simulink model "ModelRobot_NEW"  (R2020a)
settings: Solver=FixedStepDiscrete  StartTime=0.0  StopTime=30  FixedStep=0.005  RelTol=1e-3
InitFcn:
  | addpath(genpath('D:\STUDY\LVTHS_NEW\mobile-robotics-simulation-toolbox-master'))
undefined symbols (not defined in the file or in its folder): sigbuilder_block
libraries: simulink x4, mcbhostblockslib x3, mobileRoboticsLib x1
settings Model: Creator=dangh  LastModifiedBy=dangh
settings DataIOCC: ReturnWorkspaceOutputsName=out1

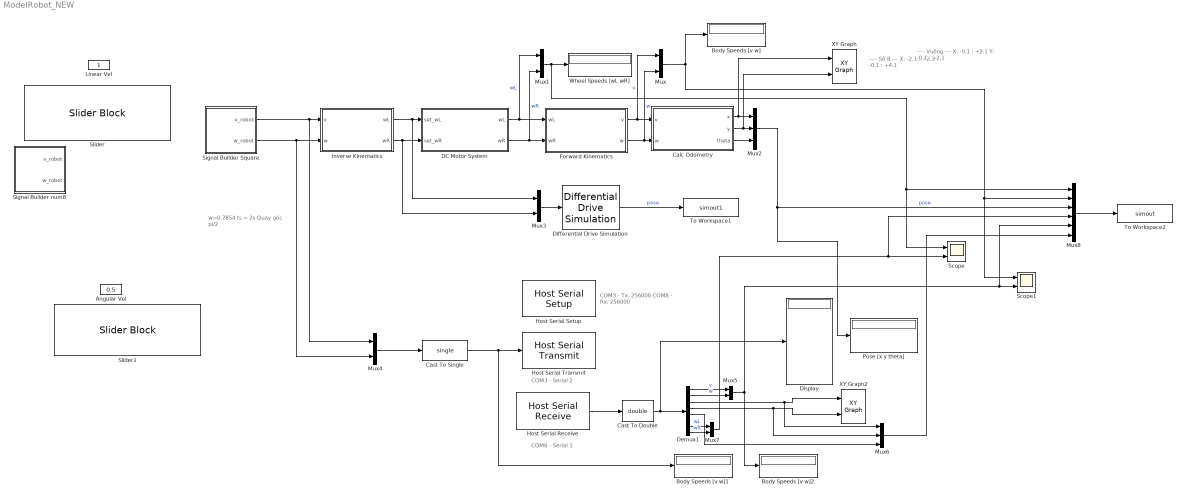
== system ModelRobot_NEW ==
  note: COM3 - Serial 2
  note: COM8 - Serial 1
  note: COM3 - Tx: 256000
      | COM8 - Rx: 256000
  note: ---- Số 8 ---
      | X: -2.1 : +2.1
      | Y: -0.1 : +4.1
  note: w=0.7854
      | ts = 2s
      | Quay góc pi/2
  note: ---- Vuông ---
      | X: -0.1 : +2.1
      | Y: -0.1 : +2.1
  Angular Vel : Constant  Value=0.5
  Body Speeds [v w] : Display
  Body Speeds [v w]1 : Display
  Body Speeds [v w]2 : Display
  Calc Odometry : MATLAB Function  TreatAsAtomicUnit=on
  Cast To Double : DataTypeConversion  OutDataTypeStr=double
  Cast To Single : DataTypeConversion  OutDataTypeStr=single
  DC Motor System : Subsystem
  Demux1 : Demux  Outputs=8
  Differential Drive Simulation : mobileRoboticsLib/Kinematic Models/Differential Drive/Differential Drive Simulation  wheelRadius=0.0625  wheelBase=0.37  initX=0  initY=0  initAngle=0  Ts=0.005
      settings: SourceProductName=Mobile Robotics Simulation Library
  Display : Display
  Forward Kinematics : MATLAB Function  TreatAsAtomicUnit=on
  Host Serial Receive : mcbhostblockslib/Host Serial Receive  serialCon=Serial 1  dataHead='S'  dataTail=0x0d  dataType=single  dataDim=8  initValue=0  errOption=Output the last received value  errValue=0  sampleTime=-1  outputStatus=off  blockingMode=off
      settings: SourceProductBaseCode=MT
  Host Serial Setup : mcbhostblockslib/Host Serial Setup  Priority=-99  comPortSer1='COM8'  baudRateA=256000  charLenA=8  stopBitA=1  parityA=none  timeoutA=1.0  ByteOrderA=LittleEndian  comPortSer2='COM3'  baudRateB=256000  charLenB=8  stopBitB=1  parityB=none  timeoutB=1.0  ByteOrderB=LittleEndian  comPortSer3='Please_select_a_port'  baudRateC=115200  charLenC=8  stopBitC=1  parityC=none  timeoutC=1.0  ByteOrderC=LittleEndian  comPortSer4='Please_select_a_port'  baudRateD=115200  charLenD=8  stopBitD=1  parityD=none  timeoutD=1.0  ByteOrderD=LittleEndian
      settings: SourceProductBaseCode=MT
  Host Serial Transmit : mcbhostblockslib/Host Serial Transmit  serialCon=Serial 2  header='S'  tail=0x0D  enableBlockingMode=off
      settings: SourceProductBaseCode=MT
  Inverse Kinematics : MATLAB Function  TreatAsAtomicUnit=on
  Linear Vel : Constant
  Mux{,1,3..5,7} (6 alike) : Mux  Inputs=2
  Mux2 : Mux  Inputs=3
  Mux6 : Mux  Inputs=3
  Mux8 : Mux  Inputs=6
  Pose [x y theta] : Display
  Scope : Scope  NumInputPorts=2
  Scope1 : Scope  NumInputPorts=2
  Signal Builder Square : Subsystem  Tag=STV Subsys  LoadFcn=sigbuilder_block('load');  StartFcn=sigbuilder_block('start');  StopFcn=sigbuilder_block('stop');  ClipboardFcn=sigbuilder_block('clipboard');  mask(Sigbuilder block){tuvar=[0:10]}
      mask help: Simulink:masks:SigbuilderBlock_MD
      mask init:
      | if ~strcmp(get_param(bdroot(gcbh),'SimulationStatus'),'stopped') tuvar = sigbuilder_block('maskInit'); end
      settings: CopyFcn=sigbuilder_block('copy');  DeleteFcn=sigbuilder_block('delete');  ModelCloseFcn=sigbuilder_block('modelClose');  PreSaveFcn=sigbuilder_block('preSave');  PauseFcn=sigbuilder_block('pause');  ContinueFcn=sigbuilder_block('continue');  NameChangeFcn=sigbuilder_block('namechange');  OpenFcn=sigbuilder_block('open',[128.25 211.5 550.5 399.75 ]);  CloseFcn=sigbuilder_block('close');
      mask Display: plot(0, 0, 100, 100,[2, 2, 32, 32, 2], [68, 8, 8, 68, 68],[32, 2], [38, 38], [32, 19, 2],[53, 60, 44], [32, 17, 17, 2],[16, 16, 31, 31]);txt = getActiveGroup(gcbh);text(2, 100, txt,'verticalAlignment', 'top');
  Signal Builder num8 : Subsystem  Tag=STV Subsys  LoadFcn=sigbuilder_block('load');  StartFcn=sigbuilder_block('start');  StopFcn=sigbuilder_block('stop');  ClipboardFcn=sigbuilder_block('clipboard');  mask(Sigbuilder block){tuvar=[0:10]}
      mask help: Simulink:masks:SigbuilderBlock_MD
      mask init:
      | if ~strcmp(get_param(bdroot(gcbh),'SimulationStatus'),'stopped') tuvar = sigbuilder_block('maskInit'); end
      settings: CopyFcn=sigbuilder_block('copy');  DeleteFcn=sigbuilder_block('delete');  ModelCloseFcn=sigbuilder_block('modelClose');  PreSaveFcn=sigbuilder_block('preSave');  PauseFcn=sigbuilder_block('pause');  ContinueFcn=sigbuilder_block('continue');  NameChangeFcn=sigbuilder_block('namechange');  OpenFcn=sigbuilder_block('open',[204 220.5 771.75 398.25 ]);  CloseFcn=sigbuilder_block('close');
      mask Display: plot(0, 0, 100, 100,[2, 2, 32, 32, 2], [68, 8, 8, 68, 68],[32, 2], [38, 38], [32, 19, 2],[53, 60, 44], [32, 17, 17, 2],[16, 16, 31, 31]);txt = getActiveGroup(gcbh);text(2, 100, txt,'verticalAlignment', 'top');
  Slider : SliderBlock  ScaleMin=-1  ScaleMax=1  TickInterval=0.25
  Slider1 : SliderBlock  ScaleMin=-1.5  ScaleMax=1.5
  To Workspace1 : ToWorkspace  VariableName=simout1  SaveFormat=Timeseries  SampleTime=-1
  To Workspace2 : ToWorkspace  VariableName=simout  SaveFormat=Timeseries  SampleTime=-1
  Wheel Speeds [wL wR] : Display
  XY Graph : simulink/Sinks/XY Graph  xmin=-2.1  xmax=2.1  ymin=-0.1  ymax=4.1  st=-1
  XY Graph2 : simulink/Sinks/XY Graph  xmin=-1  xmax=3  ymin=-2  ymax=2.5  st=-1
  wires:
  Differential Drive Simulation/1 -> To Workspace1/1  "pose"
  Inverse Kinematics/1(wL) -> DC Motor System/1(set_wL), Mux3/1
  Inverse Kinematics/2(wR) -> DC Motor System/2(set_wR), Mux3/2
  Mux/1 -> Scope1/1, Mux8/2, Body Speeds [v w]/1
  Mux1/1 -> Scope/1, Mux8/1, Wheel Speeds [wL wR]/1
  Mux3/1 -> Differential Drive Simulation/1
  DC Motor System/1(wL) -> Mux1/1, Forward Kinematics/1(wL)  "wL"
  DC Motor System/2(wR) -> Mux1/2, Forward Kinematics/2(wR)  "wR"
  Forward Kinematics/2(w) -> Mux/2, Calc Odometry/2(w)  "w"
  Forward Kinematics/1(v) -> Mux/1, Calc Odometry/1(v)  "v"
  Calc Odometry/3(theta) -> Mux2/3
  Calc Odometry/2(y) -> XY Graph/2, Mux2/2
  Calc Odometry/1(x) -> XY Graph/1, Mux2/1
  Mux2/1 -> Mux8/3, Pose [x y theta]/1  "pose"
  Mux4/1 -> Cast To Single/1
  Cast To Single/1 -> Body Speeds [v w]1/1, Host Serial Transmit/1
  Demux1/2 -> Mux5/2  "w"
  Demux1/1 -> Mux5/1  "v"
  Mux5/1 -> Mux8/5, Scope1/2, Body Speeds [v w]2/1
  Demux1/3 -> Mux6/1, XY Graph2/1
  Demux1/4 -> Mux6/2, XY Graph2/2
  Demux1/5 -> Mux6/3
  Mux6/1 -> Mux8/6
  Mux7/1 -> Mux8/4, Scope/2
  Cast To Double/1 -> Display/1, Demux1/1
  Mux8/1 -> To Workspace2/1
  Host Serial Receive/1 -> Cast To Double/1
  Signal Builder Square/2(w_robot) -> Mux4/2, Inverse Kinematics/2(w)
  Signal Builder Square/1(v_robot) -> Mux4/1, Inverse Kinematics/1(v)
  Demux1/7 -> Mux7/1  "wL"
  Demux1/8 -> Mux7/2  "wR"

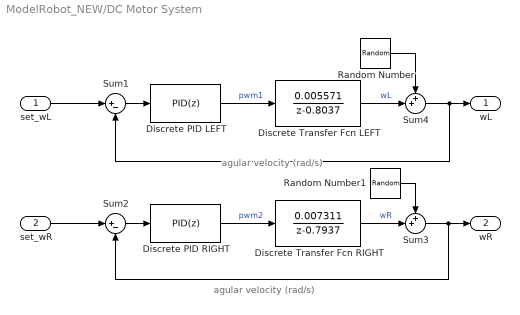
== system ModelRobot_NEW/DC Motor System ==
  note: agular velocity (rad/s)
  note: agular velocity (rad/s)
  set_wL : Inport
  set_wR : Inport  Port=2
  Discrete Transfer Fcn LEFT : DiscreteTransferFcn  Numerator=0.005571  Denominator=[1 -0.8037]
  Discrete Transfer Fcn RIGHT : DiscreteTransferFcn  Numerator=[0.007311]  Denominator=[1 -0.7937]
  Discrete PID LEFT : simulink/Continuous/PID Controller  Controller=PID  Form=Parallel  TimeDomain=Discrete-time  UseExternalTs=off  SampleTime=0.005  IntegratorMethod=Trapezoidal  FilterMethod=Forward Euler  ControllerParametersSource=internal  P=4.48920648489184  I=176.768621079225  D=0.0343896212668413  UseFilter=off  N=100  TunerSelectOption=Transfer Function Based (PID Tuner App)  InitialConditionSource=internal  InitialConditionForIntegrator=0  InitialConditionForFilter=0  DifferentiatorICPrevScaledInput=0  ExternalReset=none  TrackingMode=off  Kt=1  LimitOutput=on  UpperSaturationLimit=999  LowerSaturationLimit=-999  LinearizeAsGain=off  AntiWindupMode=none  Kb=1  POutMin=[]  POutMax=[]  IOutMin=[]  IOutMax=[]  DOutMin=[]  DOutMax=[]  NOutMin=[]  NOutMax=[]  SumOutMin=[]  SumOutMax=[]  SaturationOutMin=[]  SaturationOutMax=[]  PParamMin=[]  PParamMax=[]  IParamMin=[]  IParamMax=[]  DParamMin=[]  DParamMax=[]  NParamMin=[]  NParamMax=[]  KbParamMin=[]  KbParamMax=[]  KtParamMin=[]  KtParamMax=[]  KbOutMin=[]  KbOutMax=[]  KtOutMin=[]  KtOutMax=[]  IntegratorOutMin=[]  IntegratorOutMax=[]  FilterOutMin=[]  FilterOutMax=[]  SumI1OutMin=[]  SumI1OutMax=[]  SumI2OutMin=[]  SumI2OutMax=[]  SumI3OutMin=[]  SumI3OutMax=[]  SumI4OutMin=[]  SumI4OutMax=[]  SumDOutMin=[]  SumDOutMax=[]  DifferentiatorOutMin=[]  DifferentiatorOutMax=[]  FilterDiffOutCoefMin=[]  FilterDiffOutCoefMax=[]  ReciprocalOutMin=[]  ReciprocalOutMax=[]  SumDenOutMin=[]  SumDenOutMax=[]  SumNumOutMin=[]  SumNumOutMax=[]  DivideOutMin=[]  DivideOutMax=[]  UdiffTsProdOutMin=[]  UdiffTsProdOutMax=[]  NTsProdOutMin=[]  NTsProdOutMax=[]  UintegralTsProdOutMin=[]  UintegralTsProdOutMax=[]  UngainTsProdOutMin=[]  UngainTsProdOutMax=[]  IntegratorContinuousStateAttributes=''  IntegratorStateMustResolveToSignalObject=off  IntegratorRTWStateStorageClass=Auto  FilterContinuousStateAttributes=''  FilterStateMustResolveToSignalObject=off  FilterRTWStateStorageClass=Auto  ParallelPVariant=InternalParameters  IdealPVariant=Disabled  IVariant=InternalParameters  DVariant=InternalParameters  IntegratorVariant=Discrete  SatVariant=Enabled  AWVariant=Passthrough  PCopyVariant=Disabled  TRVariant=Disabled  FdbkBlocksVariant=Forward  IdealPFdbkVariant=Disabled  SatFdbkVariant=Disabled  DerivativeFilterVariant=Differentiator  NVariant=Passthrough  NCopyVariant=Disabled_SignalSpec  FilterICVariant=InternalICsDifferentiator  IntegratorICVariant=InternalICs  ExternalResetVariant=Disabled  TRSumVariant=Passthrough  SumFdbkVariant=Disabled  SumVariant=Sum_PID  TsampFilterVariant=InternalTs  TsampNgainVariant=Passthrough  TsampIntegralVariant=Passthrough
  Discrete PID RIGHT : simulink/Continuous/PID Controller  Controller=PID  Form=Parallel  TimeDomain=Discrete-time  UseExternalTs=off  SampleTime=0.005  IntegratorMethod=Trapezoidal  FilterMethod=Forward Euler  ControllerParametersSource=internal  P=3.42072165271296  I=141.511593847985  D=0.0251690597812978  UseFilter=off  N=100  TunerSelectOption=Transfer Function Based (PID Tuner App)  InitialConditionSource=internal  InitialConditionForIntegrator=0  InitialConditionForFilter=0  DifferentiatorICPrevScaledInput=0  ExternalReset=none  TrackingMode=off  Kt=1  LimitOutput=on  UpperSaturationLimit=999  LowerSaturationLimit=-999  LinearizeAsGain=off  AntiWindupMode=none  Kb=1  POutMin=[]  POutMax=[]  IOutMin=[]  IOutMax=[]  DOutMin=[]  DOutMax=[]  NOutMin=[]  NOutMax=[]  SumOutMin=[]  SumOutMax=[]  SaturationOutMin=[]  SaturationOutMax=[]  PParamMin=[]  PParamMax=[]  IParamMin=[]  IParamMax=[]  DParamMin=[]  DParamMax=[]  NParamMin=[]  NParamMax=[]  KbParamMin=[]  KbParamMax=[]  KtParamMin=[]  KtParamMax=[]  KbOutMin=[]  KbOutMax=[]  KtOutMin=[]  KtOutMax=[]  IntegratorOutMin=[]  IntegratorOutMax=[]  FilterOutMin=[]  FilterOutMax=[]  SumI1OutMin=[]  SumI1OutMax=[]  SumI2OutMin=[]  SumI2OutMax=[]  SumI3OutMin=[]  SumI3OutMax=[]  SumI4OutMin=[]  SumI4OutMax=[]  SumDOutMin=[]  SumDOutMax=[]  DifferentiatorOutMin=[]  DifferentiatorOutMax=[]  FilterDiffOutCoefMin=[]  FilterDiffOutCoefMax=[]  ReciprocalOutMin=[]  ReciprocalOutMax=[]  SumDenOutMin=[]  SumDenOutMax=[]  SumNumOutMin=[]  SumNumOutMax=[]  DivideOutMin=[]  DivideOutMax=[]  UdiffTsProdOutMin=[]  UdiffTsProdOutMax=[]  NTsProdOutMin=[]  NTsProdOutMax=[]  UintegralTsProdOutMin=[]  UintegralTsProdOutMax=[]  UngainTsProdOutMin=[]  UngainTsProdOutMax=[]  IntegratorContinuousStateAttributes=''  IntegratorStateMustResolveToSignalObject=off  IntegratorRTWStateStorageClass=Auto  FilterContinuousStateAttributes=''  FilterStateMustResolveToSignalObject=off  FilterRTWStateStorageClass=Auto  ParallelPVariant=InternalParameters  IdealPVariant=Disabled  IVariant=InternalParameters  DVariant=InternalParameters  IntegratorVariant=Discrete  SatVariant=Enabled  AWVariant=Passthrough  PCopyVariant=Disabled  TRVariant=Disabled  FdbkBlocksVariant=Forward  IdealPFdbkVariant=Disabled  SatFdbkVariant=Disabled  DerivativeFilterVariant=Differentiator  NVariant=Passthrough  NCopyVariant=Disabled_SignalSpec  FilterICVariant=InternalICsDifferentiator  IntegratorICVariant=InternalICs  ExternalResetVariant=Disabled  TRSumVariant=Passthrough  SumFdbkVariant=Disabled  SumVariant=Sum_PID  TsampFilterVariant=InternalTs  TsampNgainVariant=Passthrough  TsampIntegralVariant=Passthrough
  Random Number : RandomNumber  Variance=0.020583  SampleTime=0.005
  Random Number1 : RandomNumber  Variance=0.0847669  SampleTime=0.005
  Sum1 : Sum  Inputs=|+-
  Sum2 : Sum  Inputs=|+-
  Sum3 : Sum  Inputs=++|
  Sum4 : Sum  Inputs=++|
  wL : Outport
  wR : Outport  Port=2
  wires:
  Sum2/1 -> Discrete PID RIGHT/1
  Discrete PID RIGHT/1 -> Discrete Transfer Fcn RIGHT/1  "pwm2"
  set_wL/1 -> Sum1/1
  Discrete Transfer Fcn LEFT/1 -> Sum4/2  "wL"
  Sum1/1 -> Discrete PID LEFT/1
  Discrete Transfer Fcn RIGHT/1 -> Sum3/2  "wR"
  Discrete PID LEFT/1 -> Discrete Transfer Fcn LEFT/1  "pwm1"
  set_wR/1 -> Sum2/1
  Sum4/1 -> wL/1, Sum1/2
  Random Number/1 -> Sum4/1
  Random Number1/1 -> Sum3/1
  Sum3/1 -> Sum2/2, wR/1

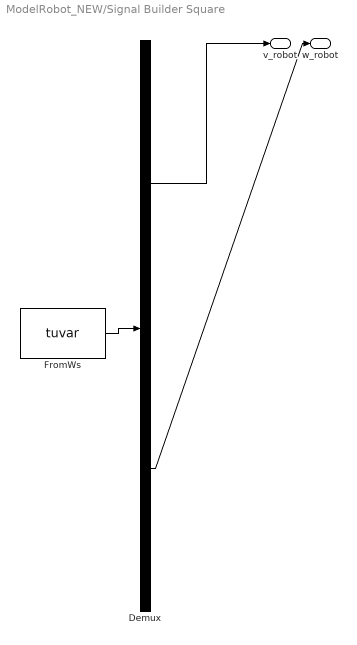
== system ModelRobot_NEW/Signal Builder Square ==
  Demux : Demux  Tag=STV Demux  Outputs=2
      settings: DisplayOption=none
  FromWs : FromWorkspace  Tag=STV FromWs  VariableName=tuvar
      SigBuilderData=|
      | common.afterFinalStr = 'Extrapolate'
      | common.sampleTime = 0
      | dataSet.timeRange = [0 30]
      | dataSet.name = 'Group 1'
      | sbobj.Groups.Name = 'Group 1'
      | sbobj.Groups.Signals(1).Name = 'v_robot'
      | sbobj.Groups.Signals(1).XData = [0 4 4 6 6 10 10 12 12 16 16 18 18 22 22 30]
      | sbobj.Groups.Signals(1).YData = [0.5 0.5 0 0 0.5 0.5 0 0 0.5 0.5 0 0 0.5 0.5 0 0]
      | sbobj.Groups.Signals(2).Name = 'w_robot'
      | sbobj.Groups.Signals(2).XData = [0 4 4 6 6 10 10 12 12 16 16 18 18 30]
      | sbobj.Groups.Signals(2).YData = [0 0 0.7854 0.7854 0 0 0.7854 0.7854 0 0 0.7854 0.7854 0 0]
      | sbobj.Groups.TimeRange = [0 30]
  v_robot : Outport  Tag=STV Outport
  w_robot : Outport  Tag=STV Outport  Port=2
  wires:
  Demux/1 -> v_robot/1
  FromWs/1 -> Demux/1
  Demux/2 -> w_robot/1

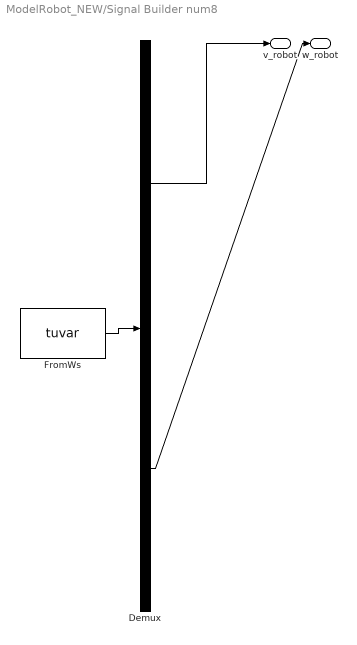
== system ModelRobot_NEW/Signal Builder num8 ==
  Demux : Demux  Tag=STV Demux  Outputs=2
      settings: DisplayOption=none
  FromWs : FromWorkspace  Tag=STV FromWs  VariableName=tuvar
      SigBuilderData=|
      | common.afterFinalStr = 'Extrapolate'
      | common.sampleTime = 0
      | dataSet.timeRange = [0 26]
      | dataSet.name = 'Group 1'
      | sbobj.Groups.Name = 'Group 1'
      | sbobj.Groups.Signals(1).Name = 'v_robot'
      | sbobj.Groups.Signals(1).XData = [0 25 25 26]
      | sbobj.Groups.Signals(1).YData = [0.5 0.5 0 0]
      | sbobj.Groups.Signals(2).Name = 'w_robot'
      | sbobj.Groups.Signals(2).XData = [0 6.283 6.283 18.849 18.849 25 25 26]
      | sbobj.Groups.Signals(2).YData = [0.5 0.5 -0.5 -0.5 0.5 0.5 0 0]
      | sbobj.Groups.TimeRange = [0 26]
  v_robot : Outport  Tag=STV Outport
  w_robot : Outport  Tag=STV Outport  Port=2
  wires:
  Demux/2 -> w_robot/1
  FromWs/1 -> Demux/1
  Demux/1 -> v_robot/1

== matlab function ModelRobot_NEW/Forward Kinematics ==
  data: v output; wL input; wR input; w output
function [v,w] = forwardKinematics(wL,wR)
    % Calculates linear and angular velocity from wheel speeds
    wheelRadius = 0.0625;
    wheelBase = 0.37;
    v = 0.5*wheelRadius*(wL+wR);
    w = (wR-wL)*wheelRadius/wheelBase;
end

== matlab function ModelRobot_NEW/Inverse Kinematics ==
  data: v input; wL output; w input; wR output
%hiennd, 04/08/2020
function [wL,wR] = inverseKinematics(v,w)   
    wheelRadius = 0.0625;
    wheelBase = 0.37;
    % Calculates wheel speeds from linear and angular velocity          
    wL = (v - w*wheelBase/2)/wheelRadius;
    wR = (v + w*wheelBase/2)/wheelRadius;
end

== matlab function ModelRobot_NEW/Calc Odometry ==
  data: v input; x output; w input; y output; theta output
function [x,y,theta] = calcOdometry(v,w)
    persistent pose
    if isempty(pose)
        pose = zeros(3,1);    % Pose matrix
    end
    sampleTime = 0.005; %5ms
    velB = [v;0;w]; % Body velocities [vx;vy;w]
    % Convert from body to world
    %theta = pose(3); == ok
    %new code
    theta = pose(3) + 0.5*w*sampleTime; %,OK, too !!!
    vel = [cos(theta) -sin(theta) 0; sin(theta) cos(theta) 0;0 0 1]*velB; 

    % Perform forward discrete integration step
    pose = pose + vel*sampleTime;
    %result
    x = pose(1);
    y = pose(2);
    theta = pose(3);
end
